simulink model "Multistring_inverter_old"  (R2025b)
settings: Solver=ode1  StartTime=0.0  StopTime=Ttotal  FixedStep=Tsample  MaxStep=1e-3  RelTol=1e-3
values from neighbouring files (symbols this model uses):
  A_0 = 1.5762    [System_parameters.m]
  alpha_T = 0.048/100    (= 0.00048)    [System_parameters.m]
  beta_T = -0.32/100    (= -0.0032)    [System_parameters.m]
  Cdc = Pdc/2/pi/Fb/Vdc_ref/Vdc_rip    (= 0.0106103295395)    [System_parameters.m]
  Cin = 3.3e-6    (= 3.3e-06)    [System_parameters.m]
  delta_x = 1    [modeling_control_para.m]
  Fb = 50    [System_parameters.m]
  fmpp = 2e3    (= 2000)    [modeling_control_para.m]
  Iscs = Iscs    (= 8.7)    [System_parameters.m]
  Kd0 = (alpha_1^2-2*Wn0_tf*damp0_tf*alpha_1*alpha_2+Wn0_tf^2*alpha_2^2)/K0/(alpha_1^3)    [modeling_control_para.m]
  Ki0 = Wn0_tf^2/K0/alpha_1    [modeling_control_para.m]
  Kp = -10    [modeling_control_para.m]
  Kp0 = (2*Wn0_tf*damp0_tf*alpha_1-Wn0_tf^2*alpha_2)/K0/alpha_1^2    [modeling_control_para.m]
  L = Vmpp_array *D0/delta_I_L/Fsw    (= 0.00349742222222)    [System_parameters.m]
  Np = 1    [System_parameters.m]
  qk0 = 11594    [System_parameters.m]
  Tau_d0 = alpha_2/alpha_1    [modeling_control_para.m]
  Ttotal = 1e-1    (= 0.1)    [modeling_control_para.m]
  Vdc_ref = 600    [System_parameters.m]
  Vmag = 230*sqrt(2)    [System_parameters.m]
  Voc_array = Vocs * Ns*Nss    (= 448.8)    [System_parameters.m]
  Vocs = Vocs/Ns    (= 0.623333333333)    [System_parameters.m]
libraries: slpidlib x2
settings Model: Creator=mwxiao  LastModifiedBy=carter
settings SolverCC: AlgebraicLoopSolver=TrustRegion
settings DataIOCC: LimitDataPoints=on  SaveFormat=Array  SignalLoggingSaveFormat=ModelDataLogs  ReturnWorkspaceOutputs=off  SignalLoggingName=sigsOut
settings OptimizationCC: ExpressionDepthLimit=2147483647.0  LifeSpan=inf
settings DebuggingCC: SaveWithParameterizedLinksMsg=none  UnderspecifiedInitializationDetection=Classic  MergeDetectMultiDrivingBlocksExec=none  SignalResolutionControl=TryResolveAllWithWarning  MultiTaskDSMMsg=warning  MultiTaskCondExecSysMsg=none  FcnCallInpInsideContextMsg=warning  UnconnectedInputMsg=warning  UnconnectedOutputMsg=warning  UnconnectedLineMsg=warning  StateNameClashWarn=warning  SFUnexpectedBacktrackingDiag=warning  SFNoUnconditionalDefaultTransitionDiag=warning  SFExecutionAtInitializationDiag=none  ArithmeticOperatorsInVariantConditions=warning
settings HardwareCC: ProdBitPerPointer=32.0  ProdBitPerSizeT=32.0  ProdBitPerPtrDiffT=32.0  ProdLargestAtomicFloat=None  ProdIntDivRoundTo=Undefined  ProdEndianess=Unspecified  ProdWordSize=32.0  ProdHWDeviceType=32-bit Generic  TargetUnknown=on
settings ModelReferenceCC: PropagateSignalLabelsOutOfModel=off
settings SFSimCC: SimUseLocalCustomCode=off  CustomCodeUndefinedFunction=UseInterfaceOnly
settings RTWCC: RTWUseLocalCustomCode=off  GPUComputeCapability=3.5
settings CodeAppCC: StateflowObjectComments=on
settings GRTTargetCC: TargetLangStandard=C89/C90 (ANSI)  CombineOutputUpdateFcns=off  GRTInterface=on
settings ConfigComp: CovMetricSettings=dw  CovSaveCumulativeToWorkspaceVar=on  CovSaveSingleToWorkspaceVar=on  CovExternalEMLEnable=off

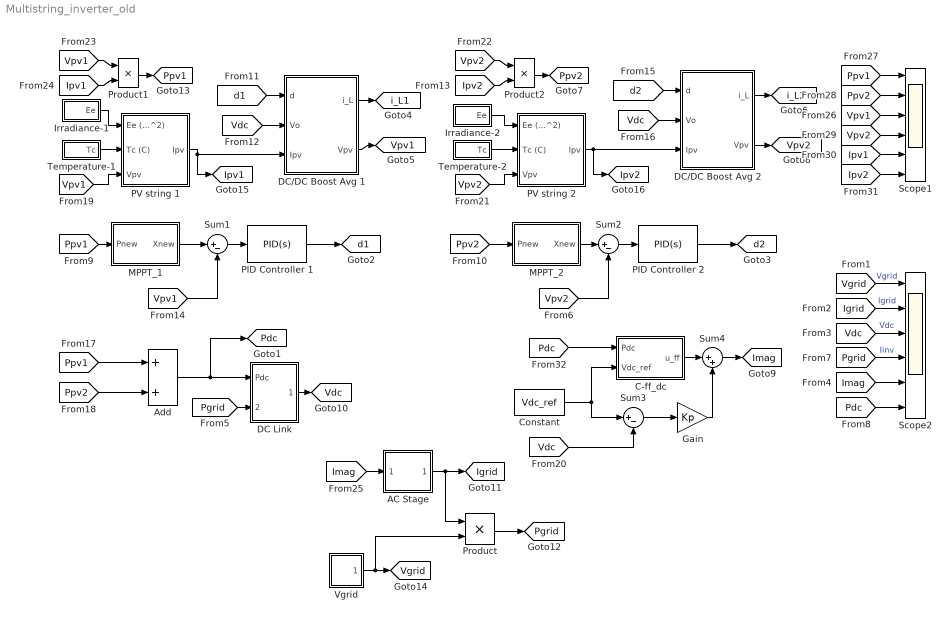
== system Multistring_inverter_old ==
  AC Stage : Subsystem
  Add : Sum
  C-ff_dc : Subsystem
  Constant : Constant  Value=Vdc_ref
  DC Link : Subsystem
  DC/DC Boost Avg 1 : Subsystem
  DC/DC Boost Avg 2 : Subsystem
  Gain : Gain  Gain=Kp
  Irradiance-1 : Subsystem
  Irradiance-2 : Subsystem
  MPPT_1 : Subsystem
  MPPT_2 : Subsystem
  PID Controller 1 : slpidlib/PID Controller  Controller=PID  Form=Parallel  TimeDomain=Continuous-time  UseExternalTs=off  SampleTime=1  IntegratorMethod=Forward Euler  FilterMethod=Forward Euler  ControllerParametersSource=internal  P=Kp0  I=Ki0  UseKiTs=off  D=Kd0  UseExternalDerivativeSource=off  N=1/Tau_d0  UseFilter=on  TunerSelectOption=Transfer Function Based (PID Tuner App)  InitialConditionSource=internal  InitialConditionForIntegrator=0  InitialConditionForFilter=0  DifferentiatorICPrevScaledInput=0  ExternalReset=none  TrackingMode=off  Kt=1  LimitOutput=on  SatLimitsSource=internal  UpperSaturationLimit=.9  LowerSaturationLimit=0  LinearizeAsGain=off  AntiWindupMode=clamping  Kb=1  LimitIntegrator=off  UpperIntegratorSaturationLimit=inf  LowerIntegratorSaturationLimit=-inf  POutMin=[]  POutMax=[]  IOutMin=[]  IOutMax=[]  DOutMin=[]  DOutMax=[]  NOutMin=[]  NOutMax=[]  SumOutMin=[]  SumOutMax=[]  SaturationOutMin=[]  SaturationOutMax=[]  PParamMin=[]  PParamMax=[]  IParamMin=[]  IParamMax=[]  DParamMin=[]  DParamMax=[]  NParamMin=[]  NParamMax=[]  KbParamMin=[]  KbParamMax=[]  KtParamMin=[]  KtParamMax=[]  KbOutMin=[]  KbOutMax=[]  KtOutMin=[]  KtOutMax=[]  IntegratorOutMin=[]  IntegratorOutMax=[]  FilterOutMin=[]  FilterOutMax=[]  SumI1OutMin=[]  SumI1OutMax=[]  SumI2OutMin=[]  SumI2OutMax=[]  SumI3OutMin=[]  SumI3OutMax=[]  SumI4OutMin=[]  SumI4OutMax=[]  SumDOutMin=[]  SumDOutMax=[]  DifferentiatorOutMin=[]  DifferentiatorOutMax=[]  FilterDiffOutCoefMin=[]  FilterDiffOutCoefMax=[]  ReciprocalOutMin=[]  ReciprocalOutMax=[]  SumDenOutMin=[]  SumDenOutMax=[]  SumNumOutMin=[]  SumNumOutMax=[]  DivideOutMin=[]  DivideOutMax=[]  UdiffTsProdOutMin=[]  UdiffTsProdOutMax=[]  NTsProdOutMin=[]  NTsProdOutMax=[]  UintegralTsProdOutMin=[]  UintegralTsProdOutMax=[]  UngainTsProdOutMin=[]  UngainTsProdOutMax=[]  ClampingZeroOutDataTypeStr=Inherit: Inherit via back propagation  ClampingZeroOutMin=[]  ClampingZeroOutMax=[]  FilterDenConstantOutDataTypeStr=Inherit: Inherit via back propagation  FilterDenConstantOutMin=[]  FilterDenConstantOutMax=[]  PCopyOutDataTypeStr=Inherit: Inherit via back propagation  PCopyOutMin=[]  PCopyOutMax=[]  NCopyOutDataTypeStr=Inherit: Inherit via back propagation  NCopyOutMin=[]  NCopyOutMax=[]  IntegratorContinuousStateAttributes=''  IntegratorStateMustResolveToSignalObject=off  IntegratorRTWStateStorageClass=Auto  FilterContinuousStateAttributes=''  FilterStateMustResolveToSignalObject=off  FilterRTWStateStorageClass=Auto  ParallelPVariant=InternalParameters  IdealPVariant=Disabled  IVariant=InternalParameters  DVariant=InternalParameters  IntegratorVariant=Continuous  SatVariant=Enabled  AWVariant=ContClampingParallel  PCopyVariant=Disabled  TRVariant=Disabled  FdbkBlocksVariant=Forward  IdealPFdbkVariant=Disabled  SatFdbkVariant=Disabled  DerivativeFilterVariant=ContFilter  NVariant=InternalParameters  NCopyVariant=Disabled  FilterICVariant=InternalICsFilter  IntegratorICVariant=InternalICs  ExternalResetVariant=Disabled  TRSumVariant=Passthrough  SumFdbkVariant=Disabled  SumVariant=Sum_PID  TsampFilterVariant=InternalTs  TsampNgainVariant=Passthrough  TsampIntegralVariant=Disabled_SignalSpec  ExternalSaturationOutDataTypeStr=Inherit: Same as second input  DerivativeSourceVariant=ErrorSignal  PreIntVariant=InternalPreInt
  PID Controller 2 : slpidlib/PID Controller  Controller=PID  Form=Parallel  TimeDomain=Continuous-time  UseExternalTs=off  SampleTime=1  IntegratorMethod=Forward Euler  FilterMethod=Forward Euler  ControllerParametersSource=internal  P=Kp0  I=Ki0  UseKiTs=off  D=Kd0  UseExternalDerivativeSource=off  N=1/Tau_d0  UseFilter=on  TunerSelectOption=Transfer Function Based (PID Tuner App)  InitialConditionSource=internal  InitialConditionForIntegrator=0  InitialConditionForFilter=0  DifferentiatorICPrevScaledInput=0  ExternalReset=none  TrackingMode=off  Kt=1  LimitOutput=on  SatLimitsSource=internal  UpperSaturationLimit=.9  LowerSaturationLimit=0  LinearizeAsGain=off  AntiWindupMode=clamping  Kb=1  LimitIntegrator=off  UpperIntegratorSaturationLimit=inf  LowerIntegratorSaturationLimit=-inf  POutMin=[]  POutMax=[]  IOutMin=[]  IOutMax=[]  DOutMin=[]  DOutMax=[]  NOutMin=[]  NOutMax=[]  SumOutMin=[]  SumOutMax=[]  SaturationOutMin=[]  SaturationOutMax=[]  PParamMin=[]  PParamMax=[]  IParamMin=[]  IParamMax=[]  DParamMin=[]  DParamMax=[]  NParamMin=[]  NParamMax=[]  KbParamMin=[]  KbParamMax=[]  KtParamMin=[]  KtParamMax=[]  KbOutMin=[]  KbOutMax=[]  KtOutMin=[]  KtOutMax=[]  IntegratorOutMin=[]  IntegratorOutMax=[]  FilterOutMin=[]  FilterOutMax=[]  SumI1OutMin=[]  SumI1OutMax=[]  SumI2OutMin=[]  SumI2OutMax=[]  SumI3OutMin=[]  SumI3OutMax=[]  SumI4OutMin=[]  SumI4OutMax=[]  SumDOutMin=[]  SumDOutMax=[]  DifferentiatorOutMin=[]  DifferentiatorOutMax=[]  FilterDiffOutCoefMin=[]  FilterDiffOutCoefMax=[]  ReciprocalOutMin=[]  ReciprocalOutMax=[]  SumDenOutMin=[]  SumDenOutMax=[]  SumNumOutMin=[]  SumNumOutMax=[]  DivideOutMin=[]  DivideOutMax=[]  UdiffTsProdOutMin=[]  UdiffTsProdOutMax=[]  NTsProdOutMin=[]  NTsProdOutMax=[]  UintegralTsProdOutMin=[]  UintegralTsProdOutMax=[]  UngainTsProdOutMin=[]  UngainTsProdOutMax=[]  ClampingZeroOutDataTypeStr=Inherit: Inherit via back propagation  ClampingZeroOutMin=[]  ClampingZeroOutMax=[]  FilterDenConstantOutDataTypeStr=Inherit: Inherit via back propagation  FilterDenConstantOutMin=[]  FilterDenConstantOutMax=[]  PCopyOutDataTypeStr=Inherit: Inherit via back propagation  PCopyOutMin=[]  PCopyOutMax=[]  NCopyOutDataTypeStr=Inherit: Inherit via back propagation  NCopyOutMin=[]  NCopyOutMax=[]  IntegratorContinuousStateAttributes=''  IntegratorStateMustResolveToSignalObject=off  IntegratorRTWStateStorageClass=Auto  FilterContinuousStateAttributes=''  FilterStateMustResolveToSignalObject=off  FilterRTWStateStorageClass=Auto  ParallelPVariant=InternalParameters  IdealPVariant=Disabled  IVariant=InternalParameters  DVariant=InternalParameters  IntegratorVariant=Continuous  SatVariant=Enabled  AWVariant=ContClampingParallel  PCopyVariant=Disabled  TRVariant=Disabled  FdbkBlocksVariant=Forward  IdealPFdbkVariant=Disabled  SatFdbkVariant=Disabled  DerivativeFilterVariant=ContFilter  NVariant=InternalParameters  NCopyVariant=Disabled  FilterICVariant=InternalICsFilter  IntegratorICVariant=InternalICs  ExternalResetVariant=Disabled  TRSumVariant=Passthrough  SumFdbkVariant=Disabled  SumVariant=Sum_PID  TsampFilterVariant=InternalTs  TsampNgainVariant=Passthrough  TsampIntegralVariant=Disabled_SignalSpec  ExternalSaturationOutDataTypeStr=Inherit: Same as second input  DerivativeSourceVariant=ErrorSignal  PreIntVariant=InternalPreInt
  PV string 1 : Subsystem
      mask Display: image(imread('icon01.jpg'))
  PV string 2 : Subsystem
      mask Display: image(imread('icon01.jpg'))
  Product : Product
  Product1 : Product  RndMeth=Zero
  Product2 : Product  RndMeth=Zero
  Scope1 : Scope  NumInputPorts=6
      settings: ActiveDisplayString=5  Title=Ipv1  ShowGrid=off  ActiveDisplayYMinimum=-2.043494935982697  ActiveDisplayYMaximum=7.4160011633406029  DataLoggingVariableName=Simout
  Scope2 : Scope  NumInputPorts=6
      settings: TimeSpan=0.03  ActiveDisplayString=6  Title=Pdc  ActiveDisplayYMinimum=-2110.0991338818271  ActiveDisplayYMaximum=5487.671251020096
  Sum1 : Sum  Inputs=|+-
  Sum2 : Sum  Inputs=|+-
  Sum3 : Sum  Inputs=|+-
  Sum4 : Sum  Inputs=|++
  Temperature-1 : Subsystem
  Temperature-2 : Subsystem
  Vgrid : Subsystem
  tag scope: Igrid=global, Imag=global, Ipv1=global, Ipv2=global, Pdc=global, Pgrid=global, Ppv1=global, Ppv2=global, Vdc=global, Vgrid=global, Vpv1=global, Vpv2=global, d1=global, d2=global, i_L1=global, i_L2=global
  wires:
  Irradiance-1/1(Ee) -> PV string 1/1(Ee (W/m^2))
  Temperature-1/1(Tc) -> PV string 1/2(Tc (C))
  [Vpv1] -> PV string 1/3(Vpv)
  Product1/1 -> [Ppv1]
  [Vpv1] -> Product1/1
  [Ipv1] -> Product1/2
  Irradiance-2/1(Ee) -> PV string 2/1(Ee (W/m^2))
  Temperature-2/1(Tc) -> PV string 2/2(Tc (C))
  [Vpv2] -> PV string 2/3(Vpv)
  PV string 2/1(Ipv) -> DC/DC Boost Avg 2/3(Ipv), [Ipv2]
  Product2/1 -> [Ppv2]
  [Vpv2] -> Product2/1
  [Ipv2] -> Product2/2
  [Vgrid] -> Scope2/1  "Vgrid"
  [Igrid] -> Scope2/2  "Igrid"
  [Vdc] -> Scope2/3  "Vdc"
  [Pgrid] -> Scope2/4  "Iinv"
  [Pdc] -> Scope2/6
  [Imag] -> Scope2/5
  [Ppv1] -> Scope1/1
  [Ppv2] -> Scope1/2
  [Vpv1] -> Scope1/3
  [Vpv2] -> Scope1/4
  [Ipv1] -> Scope1/5
  [Ipv2] -> Scope1/6
  [Pgrid] -> DC Link/2(Pinv)
  DC Link/1(Vdc) -> [Vdc]
  Add/1 -> [Pdc], DC Link/1(Pdc)
  [Ppv1] -> MPPT_1/1(Pnew)
  PID Controller 1/1 -> [d1]
  MPPT_1/1(Xnew) -> Sum1/1
  Sum1/1 -> PID Controller 1/1
  [Vpv1] -> Sum1/2
  MPPT_2/1(Xnew) -> Sum2/1
  PID Controller 2/1 -> [d2]
  [Vpv2] -> Sum2/2
  Sum2/1 -> PID Controller 2/1
  [Ppv2] -> MPPT_2/1(Pnew)
  DC/DC Boost Avg 1/2(Vpv) -> [Vpv1]
  DC/DC Boost Avg 1/1(i_L) -> [i_L1]
  [Vdc] -> DC/DC Boost Avg 1/2(Vo)
  PV string 1/1(Ipv) -> DC/DC Boost Avg 1/3(Ipv), [Ipv1]
  [d1] -> DC/DC Boost Avg 1/1(d)
  DC/DC Boost Avg 2/1(i_L) -> [i_L2]
  [d2] -> DC/DC Boost Avg 2/1(d)
  DC/DC Boost Avg 2/2(Vpv) -> [Vpv2]
  [Vdc] -> DC/DC Boost Avg 2/2(Vo)
  [Ppv1] -> Add/1
  [Ppv2] -> Add/2
  Sum4/1 -> [Imag]
  C-ff_dc/1(u_ff) -> Sum4/1
  Gain/1 -> Sum4/2
  Sum3/1 -> Gain/1
  [Vdc] -> Sum3/2
  [Pdc] -> C-ff_dc/1(Pdc)
  Constant/1 -> C-ff_dc/2(Vdc_ref), Sum3/1
  AC Stage/1(Igrid) -> Product/1, [Igrid]
  [Imag] -> AC Stage/1(Imag)
  Product/1 -> [Pgrid]
  Vgrid/1(Vgrid) -> [Vgrid], Product/2

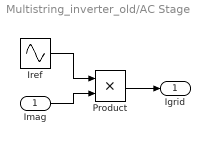
== system Multistring_inverter_old/AC Stage ==
  Imag : Inport
  Iref : Sin  Frequency=2*pi*Fb  Phase=pi/2  SampleTime=0
  Product : Product
  Igrid : Outport
  wires:
  Product/1 -> Igrid/1
  Iref/1 -> Product/1
  Imag/1 -> Product/2

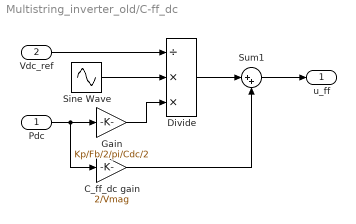
== system Multistring_inverter_old/C-ff_dc ==
  Pdc : Inport
  Vdc_ref : Inport  Port=2
  C_ff_dc gain : Gain  Gain=2/Vmag
  Divide : Product  Inputs=/**
  Gain : Gain  Gain=Kp/Fb/2/pi/Cdc/2
  Sine Wave : Sin  Amplitude=-1  Frequency=2*pi*Fb  Phase=pi/2  SampleTime=0
  Sum1 : Sum  Inputs=|++
  u_ff : Outport  SampleTime=1/fmpp
  wires:
  Sum1/1 -> u_ff/1
  Divide/1 -> Sum1/1
  Vdc_ref/1 -> Divide/1
  Sine Wave/1 -> Divide/2
  Pdc/1 -> C_ff_dc gain/1, Gain/1
  Gain/1 -> Divide/3
  C_ff_dc gain/1 -> Sum1/2

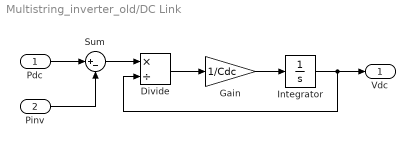
== system Multistring_inverter_old/DC Link ==
  Pdc : Inport
  Pinv : Inport  Port=2
  Divide : Product  Inputs=*/
  Gain : Gain  Gain=1/Cdc
  Integrator : Integrator  InitialCondition=Vdc_ref  LimitOutput=on  LowerSaturationLimit=0
  Sum : Sum  Inputs=|+-
  Vdc : Outport
  wires:
  Pdc/1 -> Sum/1
  Pinv/1 -> Sum/2
  Gain/1 -> Integrator/1
  Divide/1 -> Gain/1
  Sum/1 -> Divide/1
  Integrator/1 -> Divide/2, Vdc/1

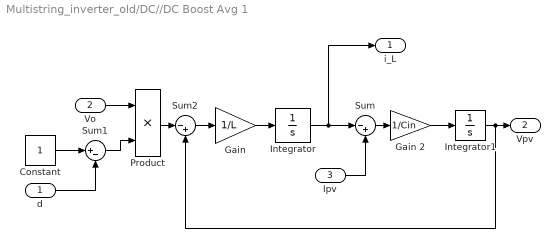
== system Multistring_inverter_old/DC//DC Boost Avg 1 ==
  d : Inport
  Vo : Inport  Port=2
  Ipv : Inport  Port=3
  Constant : Constant
  Gain : Gain  Gain=1/L
  Gain 2 : Gain  Gain=1/Cin
  Integrator : Integrator  LimitOutput=on  LowerSaturationLimit=0
  Integrator1 : Integrator  InitialCondition=Voc_array  LimitOutput=on  LowerSaturationLimit=0
  Product : Product
  Sum : Sum  Inputs=|-+
  Sum1 : Sum  Inputs=|+-
  Sum2 : Sum  Inputs=|-+
  i_L : Outport
  Vpv : Outport  Port=2
  wires:
  Gain 2/1 -> Integrator1/1
  Sum/1 -> Gain 2/1
  Ipv/1 -> Sum/2
  Integrator/1 -> i_L/1, Sum/1
  Gain/1 -> Integrator/1
  d/1 -> Sum1/2
  Sum1/1 -> Product/2
  Vo/1 -> Product/1
  Product/1 -> Sum2/1
  Sum2/1 -> Gain/1
  Integrator1/1 -> Sum2/2, Vpv/1
  Constant/1 -> Sum1/1

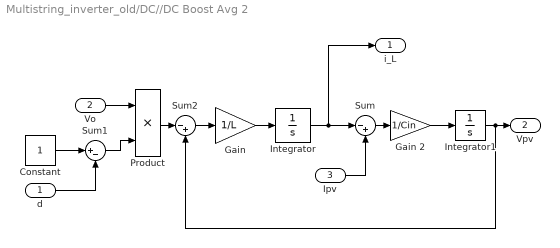
== system Multistring_inverter_old/DC//DC Boost Avg 2 ==
  d : Inport
  Vo : Inport  Port=2
  Ipv : Inport  Port=3
  Constant : Constant
  Gain : Gain  Gain=1/L
  Gain 2 : Gain  Gain=1/Cin
  Integrator : Integrator  LimitOutput=on  LowerSaturationLimit=0
  Integrator1 : Integrator  InitialCondition=Voc_array  LimitOutput=on  LowerSaturationLimit=0
  Product : Product
  Sum : Sum  Inputs=|-+
  Sum1 : Sum  Inputs=|+-
  Sum2 : Sum  Inputs=|-+
  i_L : Outport
  Vpv : Outport  Port=2
  wires:
  Gain 2/1 -> Integrator1/1
  Sum/1 -> Gain 2/1
  Ipv/1 -> Sum/2
  Integrator/1 -> i_L/1, Sum/1
  Gain/1 -> Integrator/1
  d/1 -> Sum1/2
  Sum1/1 -> Product/2
  Vo/1 -> Product/1
  Product/1 -> Sum2/1
  Sum2/1 -> Gain/1
  Integrator1/1 -> Sum2/2, Vpv/1
  Constant/1 -> Sum1/1

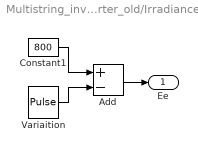
== system Multistring_inverter_old/Irradiance-1 ==
  Add : Sum  Inputs=+-
  Constant1 : Constant  Value=800
  Variaition : DiscretePulseGenerator  PulseType=Time based  Amplitude=400  Period=Ttotal  PulseWidth=50  PhaseDelay=Ttotal/2+5e-3
  Ee : Outport
  wires:
  Constant1/1 -> Add/1
  Variaition/1 -> Add/2
  Add/1 -> Ee/1

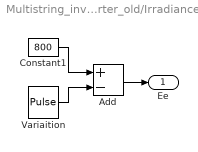
== system Multistring_inverter_old/Irradiance-2 ==
  Add : Sum  Inputs=+-
  Constant1 : Constant  Value=800
  Variaition : DiscretePulseGenerator  PulseType=Time based  Amplitude=400  Period=Ttotal  PulseWidth=50  PhaseDelay=Ttotal/2+5e-3
  Ee : Outport
  wires:
  Constant1/1 -> Add/1
  Variaition/1 -> Add/2
  Add/1 -> Ee/1

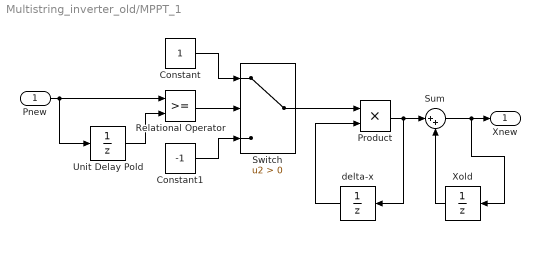
== system Multistring_inverter_old/MPPT_1 ==
  Pnew : Inport  SampleTime=1/fmpp
  Constant : Constant  SampleTime=1/fmpp
  Constant1 : Constant  Value=-1  SampleTime=1/fmpp
  Product : Product
  Relational Operator : RelationalOperator  OutDataTypeStr=boolean  RndMeth=Simplest  InputSameDT=off
  Sum : Sum  Inputs=|++
  Switch : Switch  Criteria=u2 > Threshold  SaturateOnIntegerOverflow=off  InputSameDT=off
  Unit Delay Pold : UnitDelay  InitialCondition=1e3  SampleTime=1/fmpp  HasFrameUpgradeWarning=on
  Xold : UnitDelay  InitialCondition=1e3  SampleTime=1/fmpp  HasFrameUpgradeWarning=on
  delta-x : UnitDelay  InitialCondition=delta_x  SampleTime=1/fmpp  HasFrameUpgradeWarning=on
  Xnew : Outport  SampleTime=1/fmpp
  wires:
  Pnew/1 -> Unit Delay Pold/1, Relational Operator/1
  Unit Delay Pold/1 -> Relational Operator/2
  Relational Operator/1 -> Switch/2
  Constant/1 -> Switch/1
  Constant1/1 -> Switch/3
  Switch/1 -> Product/1
  delta-x/1 -> Product/2
  Product/1 -> delta-x/1, Sum/1
  Sum/1 -> Xold/1, Xnew/1
  Xold/1 -> Sum/2

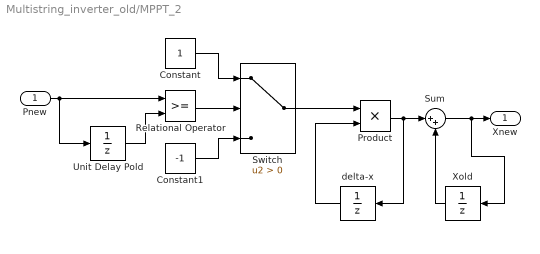
== system Multistring_inverter_old/MPPT_2 ==
  Pnew : Inport  SampleTime=1/fmpp
  Constant : Constant  SampleTime=1/fmpp
  Constant1 : Constant  Value=-1  SampleTime=1/fmpp
  Product : Product
  Relational Operator : RelationalOperator  OutDataTypeStr=boolean  RndMeth=Simplest  InputSameDT=off
  Sum : Sum  Inputs=|++
  Switch : Switch  Criteria=u2 > Threshold  SaturateOnIntegerOverflow=off  InputSameDT=off
  Unit Delay Pold : UnitDelay  InitialCondition=1e3  SampleTime=1/fmpp  HasFrameUpgradeWarning=on
  Xold : UnitDelay  InitialCondition=1e3  SampleTime=1/fmpp  HasFrameUpgradeWarning=on
  delta-x : UnitDelay  InitialCondition=delta_x  SampleTime=1/fmpp  HasFrameUpgradeWarning=on
  Xnew : Outport  SampleTime=1/fmpp
  wires:
  Pnew/1 -> Unit Delay Pold/1, Relational Operator/1
  Unit Delay Pold/1 -> Relational Operator/2
  Relational Operator/1 -> Switch/2
  Constant/1 -> Switch/1
  Constant1/1 -> Switch/3
  Switch/1 -> Product/1
  delta-x/1 -> Product/2
  Product/1 -> delta-x/1, Sum/1
  Sum/1 -> Xold/1, Xnew/1
  Xold/1 -> Sum/2

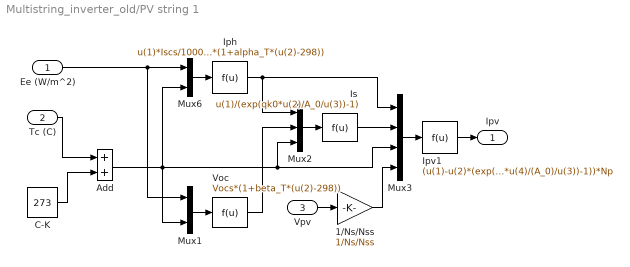
== system Multistring_inverter_old/PV string 1 ==
  Ee (W/m^2) : Inport
  Tc (C) : Inport  Port=2
  Vpv : Inport  Port=3
  1/Ns/Nss : Gain  Gain=1/Ns/Nss
  Add : Sum
  C-K : Constant  Value=273
  Iph : Fcn  Expr=u(1)*Iscs/1000*(1+alpha_T*(u(2)-298))
  Ipv1 : Fcn  Expr=(u(1)-u(2)*(exp(qk0*u(4)/(A_0)/u(3))-1))*Np
  Is : Fcn  Expr=u(1)/(exp(qk0*u(2)/A_0/u(3))-1)
  Mux1 : Mux  Inputs=2
  Mux2 : Mux  Inputs=3
  Mux3 : Mux
  Mux6 : Mux  Inputs=2
  Voc : Fcn  Expr=Vocs*(1+beta_T*(u(2)-298))
  Ipv : Outport
  wires:
  Mux6/1 -> Iph/1
  Ee (W/m^2)/1 -> Mux6/1, Mux1/1
  Mux1/1 -> Voc/1
  Mux2/1 -> Is/1
  Iph/1 -> Mux2/1, Mux3/1
  Voc/1 -> Mux2/2
  Mux3/1 -> Ipv1/1
  Is/1 -> Mux3/2
  Vpv/1 -> 1/Ns/Nss/1
  Ipv1/1 -> Ipv/1
  Tc (C)/1 -> Add/1
  Add/1 -> Mux6/2, Mux1/2, Mux3/3, Mux2/3
  C-K/1 -> Add/2
  1/Ns/Nss/1 -> Mux3/4

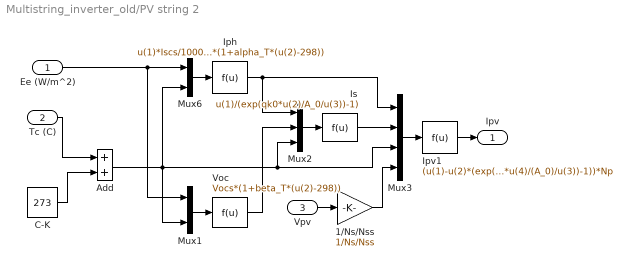
== system Multistring_inverter_old/PV string 2 ==
  Ee (W/m^2) : Inport
  Tc (C) : Inport  Port=2
  Vpv : Inport  Port=3
  1/Ns/Nss : Gain  Gain=1/Ns/Nss
  Add : Sum
  C-K : Constant  Value=273
  Iph : Fcn  Expr=u(1)*Iscs/1000*(1+alpha_T*(u(2)-298))
  Ipv1 : Fcn  Expr=(u(1)-u(2)*(exp(qk0*u(4)/(A_0)/u(3))-1))*Np
  Is : Fcn  Expr=u(1)/(exp(qk0*u(2)/A_0/u(3))-1)
  Mux1 : Mux  Inputs=2
  Mux2 : Mux  Inputs=3
  Mux3 : Mux
  Mux6 : Mux  Inputs=2
  Voc : Fcn  Expr=Vocs*(1+beta_T*(u(2)-298))
  Ipv : Outport
  wires:
  Mux6/1 -> Iph/1
  Ee (W/m^2)/1 -> Mux6/1, Mux1/1
  Mux1/1 -> Voc/1
  Mux2/1 -> Is/1
  Iph/1 -> Mux2/1, Mux3/1
  Voc/1 -> Mux2/2
  Mux3/1 -> Ipv1/1
  Is/1 -> Mux3/2
  Vpv/1 -> 1/Ns/Nss/1
  Ipv1/1 -> Ipv/1
  Tc (C)/1 -> Add/1
  Add/1 -> Mux6/2, Mux1/2, Mux3/3, Mux2/3
  C-K/1 -> Add/2
  1/Ns/Nss/1 -> Mux3/4

== system Multistring_inverter_old/Temperature-1 ==
  Add : Sum
  Constant2 : Constant  Value=28
  Variaition : DiscretePulseGenerator  PulseType=Time based  Amplitude=0  Period=20e-3  PulseWidth=50  PhaseDelay=Ttotal/4
  Tc : Outport
  wires:
  Constant2/1 -> Add/1
  Variaition/1 -> Add/2
  Add/1 -> Tc/1

== system Multistring_inverter_old/Temperature-2 ==
  Add : Sum
  Constant2 : Constant  Value=30
  Variaition : DiscretePulseGenerator  PulseType=Time based  Amplitude=0  Period=20e-3  PulseWidth=50  PhaseDelay=Ttotal/4
  Tc : Outport
  wires:
  Constant2/1 -> Add/1
  Variaition/1 -> Add/2
  Add/1 -> Tc/1

== system Multistring_inverter_old/Vgrid ==
  Product : Product
  Step1 : Step  Time=Ttotal/6+5e-3  Before=Vmag  After=Vmag  SampleTime=0
  Vgrid* : Sin  Frequency=2*pi*Fb  Phase=pi/2  SampleTime=0
  Vgrid : Outport  SampleTime=1/fmpp
  wires:
  Vgrid*/1 -> Product/1
  Step1/1 -> Product/2
  Product/1 -> Vgrid/1
